simulink model "Fly_By_Wire_Context_Diagram"  (R2024b)
settings: Solver=VariableStepAuto  StartTime=0.0  StopTime=10.0  RelTol=1e-3
settings Model: Creator=chico  LastModifiedBy=annicenajafi
settings DebuggingCC: UnderspecifiedInitializationDetection=Classic  MergeDetectMultiDrivingBlocksExec=none
settings ModelReferenceCC: PropagateSignalLabelsOutOfModel=off

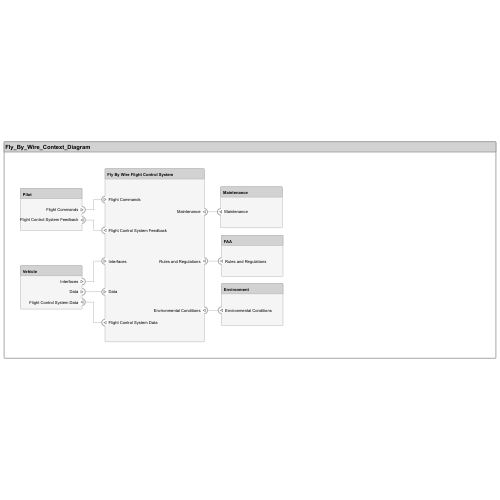
[thumbnail: Simulink's stored preview of the top-level diagram]
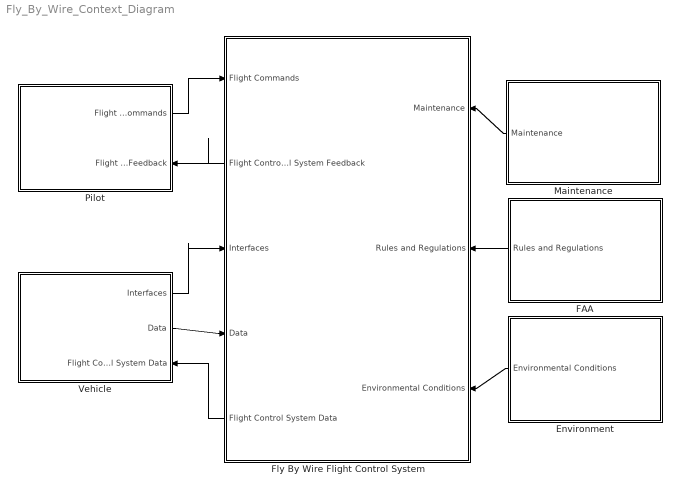
== system Fly_By_Wire_Context_Diagram ==
  Environment : Subsystem
      settings: PortSchema="{\"entries\":[{\"content\":{\"headerSize\":26,\"margin\":15,\"minimumSpacing\":25,\"sides\":[{\"content\":{\"connectorIds\":[\"Out1\"]},\"type\":\"ConnectorPlacement.EquallySpacedRectSide\",\"uuid\":\"21d662f5-504c-4947-b55b-5b7290d87f23\"},{\"content\":{\"side\":\"RIGHT\"},\"type\":\"ConnectorPlacement.EquallySpacedRectSide\",\"uuid\":\"11c8a34e-1c2d-4750-ac98-94e836f5ea6c\"},{\"content\":{\"side\":\"TOP\"},\"type\":\"ConnectorPlacement.EquallySpacedRectSide\",\"uuid\":\"378d580f-3307-4e7a-9440-aea53d895058\"}]},\"type\":\"ConnectorPlacement.EquallySpacedConnector\",\"uuid\":\"9956aad4-0c59-4231-b85e-b0aa55ff9c1b\"}],\"packageUris\":[\"http://schema.mathworks.com/mf0/Connector/R2020b\"],\"version\":\"1.0\"}"
  FAA : Subsystem
      settings: PortSchema="{\"entries\":[{\"content\":{\"headerSize\":26,\"margin\":15,\"minimumSpacing\":25,\"sides\":[{\"content\":{\"connectorIds\":[\"Out1\"]},\"type\":\"ConnectorPlacement.EquallySpacedRectSide\",\"uuid\":\"25a533d7-67e8-4107-895f-6b74cd90d28a\"},{\"content\":{\"side\":\"RIGHT\"},\"type\":\"ConnectorPlacement.EquallySpacedRectSide\",\"uuid\":\"e62c1700-ca53-407a-9d03-0af7d4700ac0\"},{\"content\":{\"side\":\"TOP\"},\"type\":\"ConnectorPlacement.EquallySpacedRectSide\",\"uuid\":\"5b20a94b-599c-4fe6-864c-4b17f05a3313\"}]},\"type\":\"ConnectorPlacement.EquallySpacedConnector\",\"uuid\":\"10c0d242-0bac-4b2f-b7cd-a6512957cf10\"}],\"packageUris\":[\"http://schema.mathworks.com/mf0/Connector/R2020b\"],\"version\":\"1.0\"}"
  Fly By Wire Flight Control System : Subsystem
      settings: PortSchema="{\"entries\":[{\"content\":{\"headerSize\":26,\"margin\":15,\"minimumSpacing\":25,\"sides\":[{\"content\":{\"connectorIds\":[\"In1\",\"Out1\",\"In5\",\"In6\",\"Out2\"]},\"type\":\"ConnectorPlacement.EquallySpacedRectSide\",\"uuid\":\"25a533d7-67e8-4107-895f-6b74cd90d28a\"},{\"content\":{\"connectorIds\":[\"In3\",\"In2\",\"In4\"],\"side\":\"RIGHT\"},\"type\":\"ConnectorPlacement.EquallySpacedRectSide\",\"uuid\":\"e62c1700-ca53-407a-9d03-0af7d4700ac0\"},{\"content\":{\"side\":\"TOP\"},\"type\":\"ConnectorPlacement.EquallySpacedRectSide\",\"uuid\":\"5b20a94b-599c-4fe6-864c-4b17f05a3313\"},{\"content\":{\"side\":\"BOTTOM\"},\"type\":\"ConnectorPlacement.EquallySpacedRectSide\",\"uuid\":\"f347d043-c667-4e93-9bdb-9cc74a2cdac7\"}]},\"type\":\"ConnectorPlacement.EquallySpacedConnector\",\"uuid\":\"10c0d242-0bac-4b2f-b7cd-a6512957cf10\"}],\"packageUris\":[\"http://schema.mathworks.com/mf0/Connector/R2020b\"],\"version\":\"1.0\"}"
  Maintenance : Subsystem
      settings: PortSchema="{\"entries\":[{\"content\":{\"headerSize\":26,\"margin\":15,\"minimumSpacing\":25,\"sides\":[{\"content\":{\"connectorIds\":[\"Out1\"]},\"type\":\"ConnectorPlacement.EquallySpacedRectSide\",\"uuid\":\"25a533d7-67e8-4107-895f-6b74cd90d28a\"},{\"content\":{\"side\":\"RIGHT\"},\"type\":\"ConnectorPlacement.EquallySpacedRectSide\",\"uuid\":\"e62c1700-ca53-407a-9d03-0af7d4700ac0\"},{\"content\":{\"side\":\"TOP\"},\"type\":\"ConnectorPlacement.EquallySpacedRectSide\",\"uuid\":\"5b20a94b-599c-4fe6-864c-4b17f05a3313\"}]},\"type\":\"ConnectorPlacement.EquallySpacedConnector\",\"uuid\":\"10c0d242-0bac-4b2f-b7cd-a6512957cf10\"}],\"packageUris\":[\"http://schema.mathworks.com/mf0/Connector/R2020b\"],\"version\":\"1.0\"}"
  Pilot : Subsystem
      settings: PortSchema="{\"entries\":[{\"content\":{\"headerSize\":26,\"margin\":15,\"minimumSpacing\":25,\"sides\":[{\"content\":{},\"type\":\"ConnectorPlacement.EquallySpacedRectSide\",\"uuid\":\"25a533d7-67e8-4107-895f-6b74cd90d28a\"},{\"content\":{\"connectorIds\":[\"Out1\",\"In1\"],\"side\":\"RIGHT\"},\"type\":\"ConnectorPlacement.EquallySpacedRectSide\",\"uuid\":\"e62c1700-ca53-407a-9d03-0af7d4700ac0\"},{\"content\":{\"side\":\"TOP\"},\"type\":\"ConnectorPlacement.EquallySpacedRectSide\",\"uuid\":\"5b20a94b-599c-4fe6-864c-4b17f05a3313\"}]},\"type\":\"ConnectorPlacement.EquallySpacedConnector\",\"uuid\":\"10c0d242-0bac-4b2f-b7cd-a6512957cf10\"}],\"packageUris\":[\"http://schema.mathworks.com/mf0/Connector/R2020b\"],\"version\":\"1.0\"}"
  Vehicle : Subsystem
      settings: PortSchema="{\"entries\":[{\"content\":{\"headerSize\":26,\"margin\":15,\"minimumSpacing\":25,\"sides\":[{\"content\":{},\"type\":\"ConnectorPlacement.EquallySpacedRectSide\",\"uuid\":\"25a533d7-67e8-4107-895f-6b74cd90d28a\"},{\"content\":{\"connectorIds\":[\"Out2\",\"Out1\",\"In1\"],\"side\":\"RIGHT\"},\"type\":\"ConnectorPlacement.EquallySpacedRectSide\",\"uuid\":\"e62c1700-ca53-407a-9d03-0af7d4700ac0\"},{\"content\":{\"side\":\"TOP\"},\"type\":\"ConnectorPlacement.EquallySpacedRectSide\",\"uuid\":\"5b20a94b-599c-4fe6-864c-4b17f05a3313\"}]},\"type\":\"ConnectorPlacement.EquallySpacedConnector\",\"uuid\":\"10c0d242-0bac-4b2f-b7cd-a6512957cf10\"}],\"packageUris\":[\"http://schema.mathworks.com/mf0/Connector/R2020b\"],\"version\":\"1.0\"}"
  wires:
  FAA/1(Rules and Regulations) -> Fly By Wire Flight Control System/2(Rules and Regulations)
  Vehicle/1(Data) -> Fly By Wire Flight Control System/6(Data)
  Pilot/1(Flight Commands) -> Fly By Wire Flight Control System/1(Flight Commands)
  Maintenance/1(Maintenance) -> Fly By Wire Flight Control System/3(Maintenance)
  Vehicle/2(Interfaces) -> Fly By Wire Flight Control System/5(Interfaces)
  Fly By Wire Flight Control System/2(Flight Control System Data) -> Vehicle/1(Flight Control System Data)
  Fly By Wire Flight Control System/1(Flight Control System Feedback) -> Pilot/1(Flight Control System Feedback)
  Environment/1(Environmental Conditions) -> Fly By Wire Flight Control System/4(Environmental Conditions)

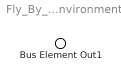
== system Fly_By_Wire_Context_Diagram/Environment ==
  Bus Element Out1 : Outport  PortName=Environmental Conditions

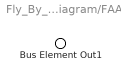
== system Fly_By_Wire_Context_Diagram/FAA ==
  Bus Element Out1 : Outport  PortName=Rules and Regulations

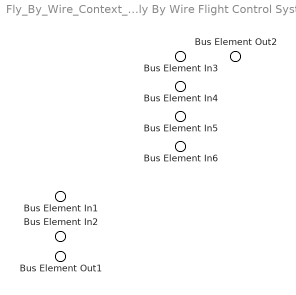
== system Fly_By_Wire_Context_Diagram/Fly By Wire Flight Control System ==
  Bus Element In3 : Inport  PortName=Flight Commands
  Bus Element In1 : Inport  Port=2  PortName=Rules and Regulations
  Bus Element In4 : Inport  Port=3  PortName=Maintenance
  Bus Element In6 : Inport  Port=4  PortName=Environmental Conditions
  Bus Element In5 : Inport  Port=5  PortName=Interfaces
  Bus Element In2 : Inport  Port=6  PortName=Data
  Bus Element Out2 : Outport  PortName=Flight Control System Feedback
  Bus Element Out1 : Outport  Port=2  PortName=Flight Control System Data

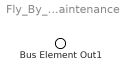
== system Fly_By_Wire_Context_Diagram/Maintenance ==
  Bus Element Out1 : Outport  PortName=Maintenance

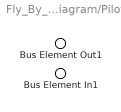
== system Fly_By_Wire_Context_Diagram/Pilot ==
  Bus Element In1 : Inport  PortName=Flight Control System Feedback
  Bus Element Out1 : Outport  PortName=Flight Commands

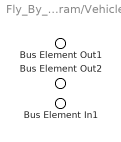
== system Fly_By_Wire_Context_Diagram/Vehicle ==
  Bus Element In1 : Inport  PortName=Flight Control System Data
  Bus Element Out1 : Outport  PortName=Data
  Bus Element Out2 : Outport  Port=2  PortName=Interfaces
